simulink model "fm_demod"  (R2018b)
settings: Solver=VariableStepAuto  StartTime=0.0  StopTime=inf  RelTol=1e-3
PreLoadFcn:
  | fs = 120e3;
  | audio_fs = 48e3;
  | [num, den] = cheby2(22,100,18e3/(fs/2),'low');
  | 
  | % nco design
  | freq_res = 0.05;                              % nco freq resolution in Hz
  | acc_wordlen = ceil(log2(1/((1/fs)*freq_res))); % calc required wordlength
  | sfdr = 80;                                  % spurious free dynamic range of nco (noise floor level)
  | phase_inc = 2^acc_wordlen/fs;    % NCO phase increment
  | quant_acc = ceil((sfdr-12)/6);          % calc number of quantised accumulator bits
  | dither_bits = ceil(acc_wordlen - quant_acc);  % calc nco dither
  | output_wordlen = 10;                                 % set op word length
  | fractional = 8;                                % set op fractional bits
undefined symbols (not defined in the file): den, dfilt, num
libraries: dspmlti4 x5, dspsigops x2, simulink x1, dspfdesign x1, sdrrlib x1, dsparch4 x1, dspobslib x1
settings Model: SimulationMode=accelerator  Creator=Tinie  LastModifiedBy=Tinie

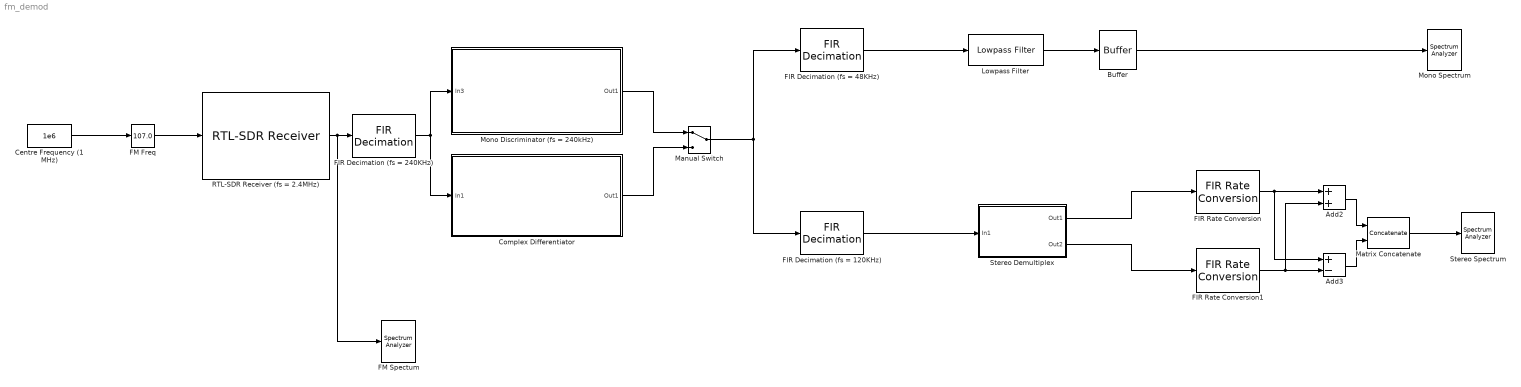
== system fm_demod ==
  Add2 : Sum
  Add3 : Sum  Inputs=+-
  Buffer : Buffer  N=4000  OutputFrames=off
  Centre Frequency (1 MHz) : Constant  Value=1e6
  Complex Differentiator : Subsystem
  FIR Decimation (fs = 120KHz) : dspmlti4/FIR Decimation  FilterSource=Dialog parameters  h=firpm(100,[0 53e3 60e3 (240e3/2)]/(240e3/2), [1 1 0 0], [1 1], 20)  D=2  filtStruct=Direct form  FilterObject=FDECIM  InputProcessing=Columns as channels (frame based)  framing=Allow multirate processing  inputOffset=0  outputBufInitCond=0  roundingMode=Floor  overflowMode=off  firstCoeffDataTypeStr=Inherit: Same word length as input  firstCoeffMin=[]  firstCoeffMax=[]  firstCoeffLastDataTypeStr=Inherit: Same word length as input  outputDataTypeStr=Inherit: Same as accumulator  outputMin=[]  outputMax=[]  outputLastDataTypeStr=Inherit: Same as accumulator
  FIR Decimation (fs = 240KHz) : dspmlti4/FIR Decimation  FilterSource=Dialog parameters  h=firpm(50,[2,120e3,240e3,(2.4e6/2)]/(2.4e6/2),[1 1 0 0], [1 1], 20)  D=10  filtStruct=Direct form  FilterObject=FDECIM  InputProcessing=Columns as channels (frame based)  framing=Allow multirate processing  inputOffset=0  outputBufInitCond=0  roundingMode=Floor  overflowMode=off  firstCoeffDataTypeStr=Inherit: Same word length as input  firstCoeffMin=[]  firstCoeffMax=[]  firstCoeffLastDataTypeStr=Inherit: Same word length as input  outputDataTypeStr=Inherit: Same as product output  outputMin=[]  outputMax=[]  outputLastDataTypeStr=Inherit: Same as product output
  "FIR Decimation (fs = 48KHz) " : dspmlti4/FIR Decimation  FilterSource=Dialog parameters  h=firpm(100,[0 15e3 20e3 (240e3/2)]/(240e3/2), [1 1 0 0], [1 1], 20)  D=5  filtStruct=Direct form  FilterObject=FDECIM  InputProcessing=Columns as channels (frame based)  framing=Allow multirate processing  inputOffset=0  outputBufInitCond=0  roundingMode=Floor  overflowMode=off  firstCoeffDataTypeStr=Inherit: Same word length as input  firstCoeffMin=[]  firstCoeffMax=[]  firstCoeffLastDataTypeStr=Inherit: Same word length as input  outputDataTypeStr=Inherit: Same as accumulator  outputMin=[]  outputMax=[]  outputLastDataTypeStr=Inherit: Same as accumulator
  FIR Rate Conversion : dspmlti4/FIR Rate Conversion  FilterSource=Dialog parameters  L=2  h=firpm(100,[0 15e3 20e3 120e3]/(120e3), [1 1 0 0], [1 1], 20)  M=5  FilterObject=FRC  roundingMode=Floor  overflowMode=off  firstCoeffDataTypeStr=Inherit: Same word length as input  firstCoeffMin=[]  firstCoeffMax=[]  firstCoeffLastDataTypeStr=Inherit: Same word length as input  outputDataTypeStr=Inherit: Same as accumulator  outputMin=[]  outputMax=[]  outputLastDataTypeStr=Inherit: Same as accumulator
      settings: SourceProductName=DSP System Toolbox  SourceProductBaseCode=DS
  FIR Rate Conversion1 : dspmlti4/FIR Rate Conversion  FilterSource=Dialog parameters  L=2  h=firpm(100,[0 15e3 20e3 240e3/2]/(240e3/2), [1 1 0 0], [1 1], 20)  M=5  FilterObject=FRC  roundingMode=Floor  overflowMode=off  firstCoeffDataTypeStr=Inherit: Same word length as input  firstCoeffMin=[]  firstCoeffMax=[]  firstCoeffLastDataTypeStr=Inherit: Same word length as input  outputDataTypeStr=Inherit: Same as accumulator  outputMin=[]  outputMax=[]  outputLastDataTypeStr=Inherit: Same as accumulator
      settings: SourceProductName=DSP System Toolbox  SourceProductBaseCode=DS
  "FM Freq " : simulink/Math Operations/Slider Gain  gain=107.0  low=94.0  high=107
  FM Spectum : SpectrumAnalyzer
  Lowpass Filter : dspfdesign/Lowpass Filter  FilterType=FIR  DesignForMinimumOrder=off  FilterOrder=50  PassbandFrequency=14.5e3  StopbandFrequency=12e3  PassbandRipple=0.2  StopbandAttenuation=50  InheritSampleRate=off  SampleRate=audio_fs  SimulateUsing=Interpreted execution  roundingMode=Floor  coeffsDataTypeStr=fixdt(1,16)
  Manual Switch : ManualSwitch
  Matrix Concatenate : Concatenate  Mode=Multidimensional array  ConcatenateDimension=2
  Mono Discriminator (fs = 240kHz) : Subsystem
  "Mono Spectrum " : SpectrumAnalyzer
  RTL-SDR Receiver (fs = 2.4MHz) : sdrrlib/RTL-SDR Receiver  IPAddress=0  CenterFrequencySource=Input port  CenterFrequency=102.5e6  GainSource=Dialog  Gain=50  ADCRate=2.4e6  FrequencyCorrection=0  LostSamplesOutputPort=off  LatencyOutputPort=off  OutputDataType=double  FrameLength=51200  EnableBurstMode=off  NumFramesInBurst=20  sobjType=sdrr.internal.SDRRTLReceiverSL  dataUDPPort=-1  ctrlUDPPort=-1  subDeviceList=nosubdev  sdrBlockType=SDRBlockTypeSLT.SDRRxBlock  requester=UNUSED_BY_SFCN  sdrExecutionMode=SDRExecutionModeSLT.ExecModeHW  BypassUserLogic=off  DecimatorSelect=DDC decimator  SourceSelect=RF data  SineAmplitude=16000  EnableInternalClock=off  BypassIQBalance=off  IFBandwidth=40e6  ADCRateSource=Dialog  IntermediateFrequency=0  DecimationFactorSource=Dialog  DecimationFactor=512  RFFrequencyIsTunable=logical(1)  SampleTime=(51200)/(2.4e6)  IFBandwidthSource=Dialog  SineFrequency=30000  BypassDCBlockingFilter=off  IntermediateFrequencySource=Dialog  IQBalanceCoefficients=64  SkipAllHardwareResetAndInitialization=off  EnableIQCalibrationTable=on  CacheIQCalibrationTable=off  EnableOffsetTuning=off  EnableRTLAGC=off  EnableTestMode=off  EnableTunerAGC=on  FrequencyCorrectionSource=Dialog  NumMLBuffers=128  NumUSBBuffers=16  RTLCrystalFrequency=28800000  TunerCrystalFrequency=28800000
      settings: SourceProductName=Communications System Toolbox Support Package for RTL-SDR Radio  SourceProductBaseCode=RTLSDR
  Stereo Demultiplex : Subsystem
  "Stereo Spectrum " : SpectrumAnalyzer
  wires:
  Centre Frequency (1 MHz)/1 -> "FM Freq "/1
  "FM Freq "/1 -> RTL-SDR Receiver (fs = 2.4MHz)/1
  RTL-SDR Receiver (fs = 2.4MHz)/1 -> FM Spectum/1, FIR Decimation (fs = 240KHz)/1
  FIR Decimation (fs = 240KHz)/1 -> Complex Differentiator/1(In1), Mono Discriminator (fs = 240kHz)/1(In3)
  FIR Rate Conversion1/1 -> Add2/2, Add3/2
  Add3/1 -> Matrix Concatenate/2
  Matrix Concatenate/1 -> "Stereo Spectrum "/1
  Add2/1 -> Matrix Concatenate/1
  FIR Rate Conversion/1 -> Add3/1, Add2/1
  FIR Decimation (fs = 120KHz)/1 -> Stereo Demultiplex/1(In1)
  Stereo Demultiplex/1(Out1) -> FIR Rate Conversion/1
  Stereo Demultiplex/2(Out2) -> FIR Rate Conversion1/1
  "FIR Decimation (fs = 48KHz) "/1 -> Lowpass Filter/1
  Lowpass Filter/1 -> Buffer/1
  Buffer/1 -> "Mono Spectrum "/1
  Manual Switch/1 -> "FIR Decimation (fs = 48KHz) "/1, FIR Decimation (fs = 120KHz)/1
  Mono Discriminator (fs = 240kHz)/1(Out1) -> Manual Switch/1
  Complex Differentiator/1(Out1) -> Manual Switch/2

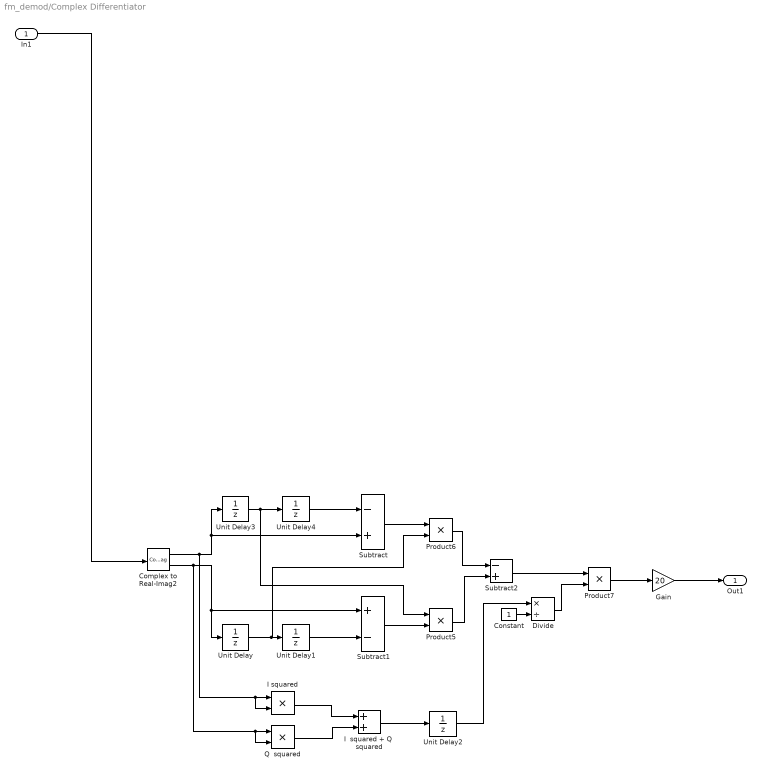
== system fm_demod/Complex Differentiator ==
  In1 : Inport
  Complex to Real-Imag2 : ComplexToRealImag
  Constant : Constant
  Divide : Product  Inputs=*/
  Gain : Gain  Gain=20
  I  squared + Q  squared : Sum
  I squared : Product
  Product5 : Product
  Product6 : Product
  Product7 : Product
  Q  squared : Product
  Subtract : Sum  Inputs=-+
  Subtract1 : Sum  Inputs=+-
  Subtract2 : Sum  Inputs=-+
  Unit Delay{,1..4} (5 alike) : UnitDelay  SampleTime=-1
  Out1 : Outport
  wires:
  Product5/1 -> Subtract2/2
  Unit Delay3/1 -> Unit Delay4/1, Product5/1
  Product6/1 -> Subtract2/1
  Subtract2/1 -> Product7/1
  Divide/1 -> Product7/2
  Complex to Real-Imag2/2 -> Q  squared/2, Q  squared/1, Unit Delay/1, Subtract1/1
  Unit Delay4/1 -> Subtract/1
  I squared/1 -> I  squared + Q  squared/1
  Complex to Real-Imag2/1 -> I squared/2, I squared/1, Unit Delay3/1, Subtract/2
  Unit Delay/1 -> Product6/2, Unit Delay1/1
  Constant/1 -> Divide/2
  Subtract1/1 -> Product5/2
  Q  squared/1 -> I  squared + Q  squared/2
  Subtract/1 -> Product6/1
  Unit Delay1/1 -> Subtract1/2
  I  squared + Q  squared/1 -> Unit Delay2/1
  Unit Delay2/1 -> Divide/1
  In1/1 -> Complex to Real-Imag2/1
  Product7/1 -> Gain/1
  Gain/1 -> Out1/1

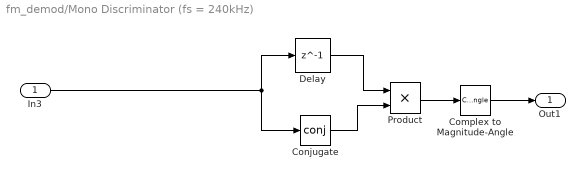
== system fm_demod/Mono Discriminator (fs = 240kHz) ==
  In3 : Inport
  Complex to Magnitude-Angle : ComplexToMagnitudeAngle  Output=Angle
  Conjugate : Math  Operator=conj  SaturateOnIntegerOverflow=on
  Delay : Delay  DelayLength=1  InputProcessing=Columns as channels (frame based)
  Product : Product
  Out1 : Outport
  wires:
  Conjugate/1 -> Product/2
  In3/1 -> Delay/1, Conjugate/1
  Product/1 -> Complex to Magnitude-Angle/1
  Delay/1 -> Product/1
  Complex to Magnitude-Angle/1 -> Out1/1

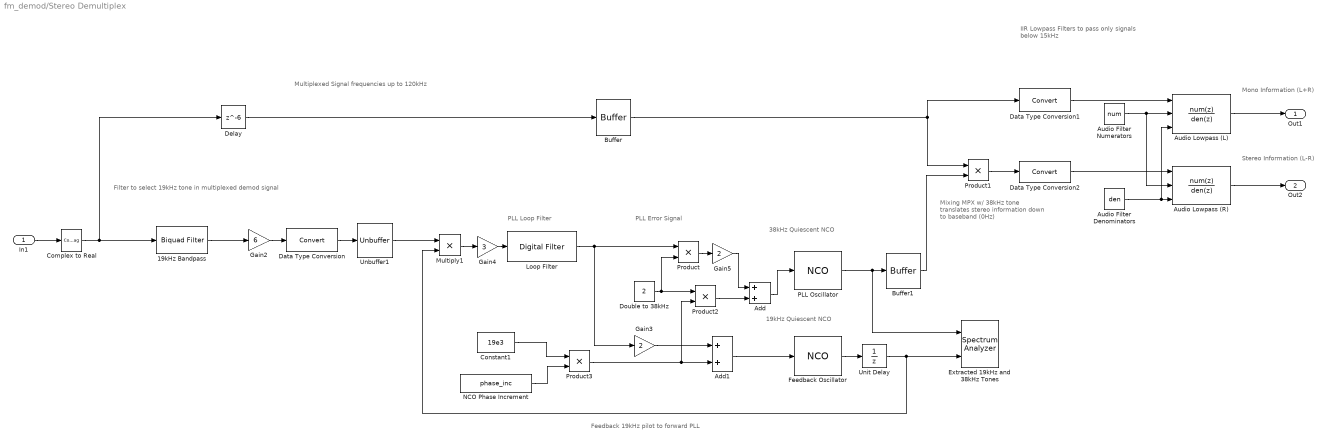
== system fm_demod/Stereo Demultiplex ==
  note: Mixing MPX w/ 38kHz tone translates stereo information down to baseband (0Hz)
  note: Mono Information (L+R)
  note: Multiplexed Signal frequencies up to 120kHz
  note: Filter to select 19kHz tone in multiplexed demod signal
  note: PLL Error Signal
  note: IIR Lowpass Filters to pass only signals below 15kHz
  note: 38kHz Quiescent NCO
  note: 19kHz Quiescent NCO
  note: Feedback 19kHz pilot to forward PLL
  note: PLL Loop Filter
  note: Stereo Information (L-R)
  In1 : Inport
  19kHz Bandpass : dsparch4/Biquad Filter  Tag=BlockMethodSubSystem  FilterSource=Dialog parameters  CoeffSource=Specify via dialog  FilterObject=dfilt.df2tsos([1 0.3 0.4],[1 0.1 0.2])  IIRFiltStruct=Direct form II  BiQuadCoeffs=[0.0083392806558967407 -0.016678561311793474 0.0083392806558967355 1 -1.0916485720976647 0.99738928062166954;0.0030175126661685031 0 -0.0030175126661685031 1 -1.0840484113399906 0.99738159148297845;0.32375855758621658 0.64751711517243304 0.32375855758621636 1 -1.0864337865299356 0.9947776723347781]  ScaleValues=[0.002190967548082783;1;1;1]  IC=0  ICnum=0  ICden=0  a0Flag=Warning  optimizeScaleValues=off  ScaleValueMode=Specify via input port (g)  InputProcessing=Columns as channels (frame based)  roundingMode=Floor  overflowMode=off  scaleValueFracLength=14  denProdOutputFracLength=30  denAccumFracLength=30  secondMemoryFracLength=15
      settings: SourceProductName=DSP System Toolbox
  Add : Sum  OutDataTypeStr=Inherit: Same as first input
  Add1 : Sum  OutDataTypeStr=Inherit: Same as first input
  Audio Filter Denominators : Constant  Value=den
  "Audio Filter Numerators " : Constant  Value=num
  Audio Lowpass (L) : DiscreteFilter  NumeratorSource=Input port  Numerator=[0.5 0.5]  DenominatorSource=Input port  Denominator=[1 0.1]  InputProcessing=Columns as channels (frame based)  FilterStructure=Direct form II transposed  a0EqualsOne=on
      settings: InputPortMap=u0,p1,p3
  Audio Lowpass (R) : DiscreteFilter  NumeratorSource=Input port  Numerator=[0.5 0.5]  DenominatorSource=Input port  Denominator=[1 0.1]  InputProcessing=Columns as channels (frame based)  FilterStructure=Direct form II transposed  a0EqualsOne=on
      settings: InputPortMap=u0,p1,p3
  Buffer : Buffer  N=4000  OutputFrames=off
  Buffer1 : Buffer  N=4000  OutputFrames=off
  Complex to Real : ComplexToRealImag  Output=Real
  Constant1 : Constant  Value=19e3  OutDataTypeStr=uint32
  Data Type Conversion : DataTypeConversion  RndMeth=Zero
  Data Type Conversion1 : DataTypeConversion  RndMeth=Simplest
  Data Type Conversion2 : DataTypeConversion  RndMeth=Simplest
  Delay : Delay  DelayLength=6  InitialCondition=0  InputProcessing=Columns as channels (frame based)
  Double to 38kHz : Constant  Value=2
  "Extracted 19kHz and 38kHz Tones " : SpectrumAnalyzer  NumInputPorts=2
  Feedback Oscillator : dspsigops/NCO  AccIncSrc=Input port  AccInc=100  PhaseOffsetSrc=Specify via dialog  PhaseOffset=0  AccumWL=acc_wordlen  HasDither=on  DitherWL=dither_bits  PNgeneratorLength=19  HasPhaseQuantizer=on  TableDepth=quant_acc  HasOutputPhaseError=off  Formula=Cosine  DataType=Binary point scaling  OutputWL=output_wordlen  OutputFL=fractional  CompMethod=Table lookup (no interpolation)  SampleTime=1  SamplesPerFrame=1  OutputFrames=off
      settings: SourceProductName=DSP System Toolbox  SourceProductBaseCode=DS
  Gain2 : Gain  Gain=6
  Gain3 : Gain  Gain=2  OutDataTypeStr=int32
  Gain4 : Gain  Gain=3
  Gain5 : Gain  Gain=2  OutDataTypeStr=int32
  Loop Filter : dspobslib/Digital Filter  TypePopup=IIR (poles & zeros)  IIRFiltStruct=Direct form II transposed  AllPoleFiltStruct=Direct form  FIRFiltStruct=Direct form  CoeffSource=Specify via dialog  NumCoeffs=[0,1,-0.994711805058698]  DenCoeffs=[1,-1.96959417190845,0.969594171908450]  BiQuadCoeffs=[1 0.3 0.4 1 0.1 0.2]  LatticeCoeffs=[0.2 0.4]  denIgnore=on  FiltPerSampPopup=One filter per frame  IC=0  ICnum=0  ICden=0  roundingMode=Nearest  overflowMode=off  ScaleValues=1  scaleValueFracLength=14  stageInFracLength=15  stageOutFracLength=15  FilterSource=Specify via dialog  dfiltObjectName=dfilt.dffir([1 2 1])  InputProcessing=Inherited (this choice will be removed - see release notes)
      settings: SourceProductName=DSP System Toolbox  SourceProductBaseCode=DS
  Multiply1 : Product  OutDataTypeStr=Inherit: Inherit via back propagation
  NCO Phase Increment : Constant  Value=phase_inc  OutDataTypeStr=uint32
  PLL Oscillator : dspsigops/NCO  AccIncSrc=Input port  AccInc=100  PhaseOffsetSrc=Specify via dialog  PhaseOffset=0  AccumWL=acc_wordlen  HasDither=on  DitherWL=dither_bits  PNgeneratorLength=19  HasPhaseQuantizer=on  TableDepth=quant_acc  HasOutputPhaseError=off  Formula=Cosine  DataType=Binary point scaling  OutputWL=output_wordlen  OutputFL=fractional  CompMethod=Table lookup (no interpolation)  SampleTime=1  SamplesPerFrame=1  OutputFrames=off
      settings: SourceProductName=DSP System Toolbox  SourceProductBaseCode=DS
  Product : Product
  Product1 : Product
  Product2 : Product
  Product3 : Product  OutDataTypeStr=Inherit: Same as first input
  Unbuffer1 : Unbuffer
  Unit Delay : UnitDelay  SampleTime=-1
  Out1 : Outport
  Out2 : Outport  Port=2
  wires:
  Audio Lowpass (R)/1 -> Out2/1
  Delay/1 -> Buffer/1
  Data Type Conversion1/1 -> Audio Lowpass (L)/1
  Product/1 -> Gain5/1
  Product1/1 -> Data Type Conversion2/1
  Complex to Real/1 -> Delay/1, 19kHz Bandpass/1
  Audio Filter Denominators/1 -> Audio Lowpass (L)/3, Audio Lowpass (R)/3
  Constant1/1 -> Product3/1
  Gain4/1 -> Loop Filter/1
  Product2/1 -> Add/2
  Buffer/1 -> Data Type Conversion1/1, Product1/1
  Buffer1/1 -> Product1/2
  Loop Filter/1 -> Product/1, Gain3/1
  Gain5/1 -> Add/1
  PLL Oscillator/1 -> "Extracted 19kHz and 38kHz Tones "/1, Buffer1/1
  "Audio Filter Numerators "/1 -> Audio Lowpass (R)/2, Audio Lowpass (L)/2
  Double to 38kHz/1 -> Product2/1, Product/2
  Multiply1/1 -> Gain4/1
  19kHz Bandpass/1 -> Gain2/1
  Product3/1 -> Product2/2, Add1/2
  Add1/1 -> Feedback Oscillator/1
  Feedback Oscillator/1 -> Unit Delay/1
  Add/1 -> PLL Oscillator/1
  Gain3/1 -> Add1/1
  Gain2/1 -> Data Type Conversion/1
  Unbuffer1/1 -> Multiply1/1
  Data Type Conversion/1 -> Unbuffer1/1
  Data Type Conversion2/1 -> Audio Lowpass (R)/1
  NCO Phase Increment/1 -> Product3/2
  Unit Delay/1 -> "Extracted 19kHz and 38kHz Tones "/2, Multiply1/2
  Audio Lowpass (L)/1 -> Out1/1
  In1/1 -> Complex to Real/1
